simulink model "robio_auv5dof2017b"  (R2018b)
settings: Solver=VariableStepAuto  StartTime=0.0  StopTime=8.0  RelTol=0.05
settings Model: Creator=aditya-ubuntu  LastModifiedBy=aditya-ubuntu
settings SolverCC: MaxConsecutiveMinStep=10  MinimalZcImpactIntegration=on
settings DebuggingCC: ReadBeforeWriteMsg=DisableAll  WriteAfterWriteMsg=DisableAll  WriteAfterReadMsg=DisableAll  MultiTaskDSMMsg=none  UnderSpecifiedDimensionMsg=error
settings ModelReferenceCC: UpdateModelReferenceTargets=IfOutOfDate
settings SFSimCC: SFSimEcho=off

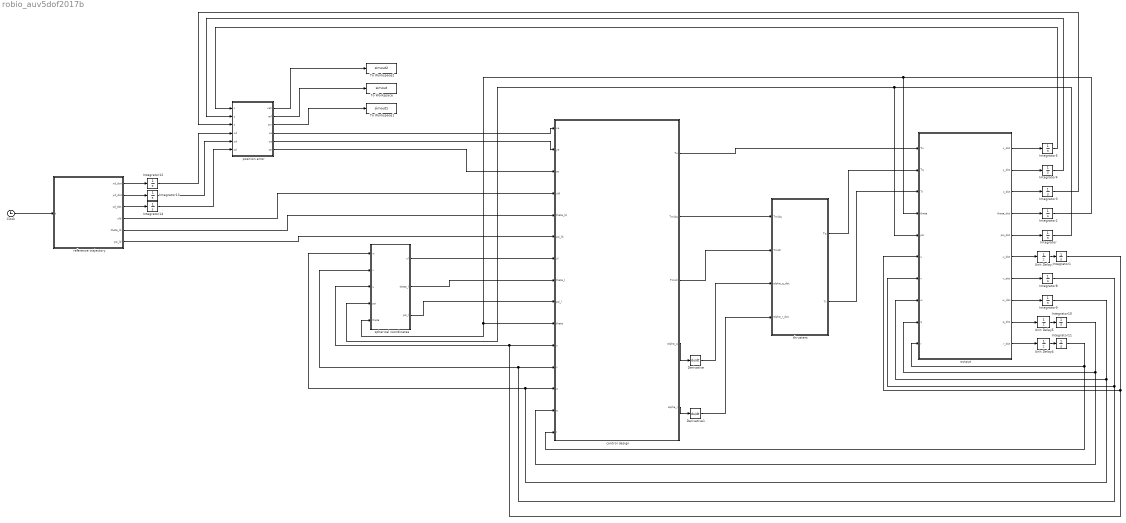
== system robio_auv5dof2017b ==
  Clock : Clock
      settings: Decimation=100
  Derivative : Derivative
  Derivative1 : Derivative
  Integrator{,2,4,8..9,12} (6 alike) : Integrator
  Integrator1 : Integrator  InitialCondition=0.3  AbsoluteTolerance=0.05
  Integrator10 : Integrator  InitialCondition=0.00001
  Integrator11 : Integrator  InitialCondition=0.0000001  AbsoluteTolerance=0.05
  Integrator13 : Integrator  InitialCondition=20
  Integrator14 : Integrator  InitialCondition=5
  Integrator3 : Integrator  InitialCondition=10
  Integrator5 : Integrator  InitialCondition=10
  To Workspace : ToWorkspace  VariableName=simout  SaveFormat=Timeseries  SampleTime=-1
  To Workspace1 : ToWorkspace  VariableName=simout1  SaveFormat=Timeseries  SampleTime=-1
  To Workspace2 : ToWorkspace  VariableName=simout2  SaveFormat=Timeseries  SampleTime=-1
  Unit Delay3 : UnitDelay  SampleTime=-1
  Unit Delay4 : UnitDelay  SampleTime=-1
  Unit Delay5 : UnitDelay  SampleTime=-1
  control design : MATLAB Function  TreatAsAtomicUnit=on
  output : MATLAB Function  TreatAsAtomicUnit=on
  position error : MATLAB Function  TreatAsAtomicUnit=on
  reference trajectory : MATLAB Function  TreatAsAtomicUnit=on
  spherical coordinates : MATLAB Function  TreatAsAtomicUnit=on
  thrusters : MATLAB Function  TreatAsAtomicUnit=on
  wires:
  output/1(x_dot) -> Integrator5/1
  output/2(y_dot) -> Integrator4/1
  output/3(z_dot) -> Integrator3/1
  output/4(theta_dot) -> Integrator2/1
  output/5(psi_dot) -> Integrator/1
  output/6(u_dot) -> Unit Delay3/1
  Integrator5/1 -> position error/1(x)
  Integrator4/1 -> position error/2(y)
  output/7(v_dot) -> Integrator8/1
  output/8(w_dot) -> Integrator9/1
  output/9(q_dot) -> Unit Delay5/1
  Integrator10/1 -> output/9(q), control design/14(q)
  Integrator9/1 -> output/8(w), spherical coordinates/1(w), control design/13(w)
  Integrator8/1 -> output/7(v), spherical coordinates/2(v), control design/12(v)
  Integrator1/1 -> output/6(u), spherical coordinates/3(u), control design/11(u)
  Integrator/1 -> output/5(psi), spherical coordinates/4(psi)
  Integrator2/1 -> output/4(theta), spherical coordinates/5(theta), control design/10(theta)
  Integrator11/1 -> control design/15(r), output/10(r)
  spherical coordinates/2(theta_l) -> control design/8(theta_l)
  spherical coordinates/3(psi_l) -> control design/9(psi_l)
  spherical coordinates/1(ul) -> control design/7(ul)
  reference trajectory/4(uld) -> control design/4(uld)
  Integrator3/1 -> position error/3(z)
  Unit Delay3/1 -> Integrator1/1
  Unit Delay4/1 -> Integrator11/1
  output/10(r_dot) -> Unit Delay4/1
  position error/6(ze) -> control design/3(ze)
  reference trajectory/1(xd_dot) -> Integrator12/1
  reference trajectory/2(yd_dot) -> Integrator13/1
  reference trajectory/3(zd_dot) -> Integrator14/1
  position error/5(ye) -> control design/2(ye)
  Integrator13/1 -> position error/5(yd)
  Integrator12/1 -> position error/4(xd)
  Integrator14/1 -> position error/6(zd)
  Unit Delay5/1 -> Integrator10/1
  position error/2(ref) -> To Workspace/1
  position error/3(err) -> To Workspace1/1
  position error/4(xe) -> control design/1(xe)
  position error/1(veh) -> To Workspace2/1
  reference trajectory/5(theta_ld) -> control design/5(theta_ld)
  reference trajectory/6(psi_ld) -> control design/6(psi_ld)
  Clock/1 -> reference trajectory/1(t)
  control design/2(Tmidq) -> thrusters/1(Tmidq)
  control design/3(Tmidr) -> thrusters/2(Tmidr)
  control design/4(alpha_q) -> Derivative/1
  control design/5(alpha_r) -> Derivative1/1
  thrusters/1(Tq) -> output/2(Tq)
  thrusters/2(Tr) -> output/3(Tr)
  Derivative/1 -> thrusters/3(alpha_q_dot)
  Derivative1/1 -> thrusters/4(alpha_r_dot)
  control design/1(Tu) -> output/1(Tu)

== matlab function robio_auv5dof2017b/thrusters ==
  data: Tq output; Tr output; Tmidq input; Tmidr input; alpha_q_dot input; alpha_r_dot input
function [Tq, Tr] = fcn(Tmidq, Tmidr, alpha_q_dot, alpha_r_dot)

    m5 = 22.5;
    m6 = 15.0;
    
%     disp('Tmidq');
%     disp(Tmidq);
%     disp('Tmidr');
%     disp(Tmidr);
%     disp('alpha_q_dot');
%     disp(alpha_q_dot);
%     disp('alpha_r_dot');
%     disp(alpha_r_dot);
    
    Tq = m5*( Tmidq + alpha_q_dot);
    
    disp("Tq");
    disp(Tq);
    
    Tr = m6*( Tmidr + alpha_r_dot);
    
    disp("Tr");
    disp(Tr);
       
end

== matlab function robio_auv5dof2017b/control design ==
  data: Tu output; Tmidq output size=6; Tmidr output; xe input; ye input size=3; ze input; uld input; theta_ld input; psi_ld input; ul input; theta_l input; psi_l input; theta input; u input; v input; w input; q input; r input; alpha_q output; alpha_r output
function [Tu, Tmidq, Tmidr, alpha_q, alpha_r] = controlinputfn5dof(xe, ye, ze, uld, theta_ld, psi_ld, ul, theta_l, psi_l, theta, u, v, w, q, r)
    
    gamma_r = 1.2;
    gamma_q = 1.2;
    gamma_u = 1;
    gamma_psi = 0.6;
    gamma_theta = 0.6;
    gamma_re = 1.2;
    
    k_psi = 0.5;
    k_theta = 0.5;
    k_u = 12;
    k_r = 0.9;
    k_q = 0.9;
    c_theta = 0.5;
    c_u = 12;
    
    m = [ 25.0 17.5 30.0 1.0 22.5 15.0 ];
    onebym = [1/25.0 1/17.5 1/30.0 1.0 1/22.5 1/15.0];
    row_g_invtri_Gml = 5.0;
    
    fu = (m(2)*v*r*onebym(1)) - (m(3)*w*q*onebym(1));    
    fv = (-(m(1)*u*r*onebym(2)));    
    fw = (m(1)*u*q*onebym(3));    
    fq = ((m(3)-m(1))*u*w*onebym(5)) - ((row_g_invtri_Gml)*onebym(5)*sin(theta));    
    fr = (m(1)-m(2))*u*v*onebym(6);
    
    disp('xe');
    disp(xe);
    disp('ye');
    disp(ye);
    disp('ze');
    disp(ze);
    
    re = sqrt(xe^2 + ye^2 + ze^2);
    
    disp('re');
    disp(re);
    xe_dot = uld*cos(theta_ld)*cos(psi_ld) - ul*cos(theta_l)*cos(psi_l);
    ye_dot = uld*cos(theta_ld)*sin(psi_ld) - ul*cos(theta_l)*sin(psi_l);
    ze_dot = -uld*sin(theta_ld) + ul*sin(theta_l);
    
    disp('xe_dot');
    disp(xe_dot);
    disp('ye_dot');
    disp(xe_dot);
    disp('ze_dot');
    disp(xe_dot);

    theta_a = atan2(w,sqrt(u^2 + v^2));
    theta_b = atan2( ze, sqrt(xe^2 + ye^2) );
    theta_le = theta_b - theta_l;
   
    psi_a = atan2(v,u);
    psi_b = atan2(ye,xe);
    psi_le = psi_b - psi_l;
    
    epower = e^(-c_theta*re);
    
    angle_in = (theta_ld - theta_b)*epower;
    
    uld_m = uld + c_u*re*cos(angle_in);
        
    theta_ld_m = theta_b + angle_in;
    
    re_dot = uld*{ cos(theta_ld)*cos(theta_b) + sin(theta_ld)*sin(theta_b)} - ul*{ cos(theta_l)*cos(theta_b)*cos(psi_le) + sin(theta_l)*sin(theta_b) };
    
    theta_b_dot = ((xe^2 + ye^2)*ze_dot - ze*(xe*xe_dot + ye*ye_dot)) / (re*re*sqrt(xe^2+ye^2));
    
    uld_m_dot = c_u*re_dot*cos(angle_in) - {c_u*re*epower*(theta_b*c_theta*re*re_dot - theta_b_dot)*sin(angle_in)};
    
    theta_ld_m_dot = theta_b_dot*(1 - epower) - c_theta*re*angle_in;
    
    ule = uld_m - ul;
    
    psi_b_dot = ( xe*ye_dot - ye*xe_dot ) / ( xe^2 + ye^2 );
    
    % duc*T is ignored
    Tu = m(1)*sec(theta_a)*sec(psi_a)*{ gamma_u^(-1)*{ k_u*ule + re*cos(theta_ld_m - theta_b)} +  uld_m_dot - fv*cos(theta_a)*sin(psi_a) - fw*sin(theta_a) };
    disp("Tu");
    disp(Tu);
    
    theta_leby2 = theta_le/2;
    theta_leby2_inv = 2/theta_le;
    theta_frac = (theta_ld_m + theta_l)/2;
    
    % dqc*T is ignored
    alpha_q_part1 = gamma_theta^(-1)*{ k_theta*theta_le - gamma_re^(-1)*re*ul*sin(theta_frac - theta_b)*sin(theta_leby2)*(theta_leby2_inv) };       
    alpha_q_part2 = theta_ld_m_dot + ( fw*(u^2 + v^2) - w*u*(fu + m(1)*Tu) + v*fv )/( ul*sqrt(u^2 + v^2) );    
    alpha_q = alpha_q_part1 + alpha_q_part2;
    disp('alpha_q');
    disp(alpha_q);
    eq = alpha_q - q;
    
    % drc*T is ignored
    alpha_r = cos(theta)*{ gamma_psi^(-1)*k_psi*psi_le + psi_b_dot - ( (u*fu - v(fu + m(1)*Tu))/ (u^2+v^2) ) };
    disp('alpha_r');
    disp(alpha_r);
    er = alpha_r - r;
    
   
    Tmidq = gamma_q^(-1)*(k_q*eq - gamma_theta*theta_le) - fq;
    disp("Tq");
    disp(Tq);
        
    Tmidr = gamma_r^(-1)*(k_r*er - gamma_psi*psi_le*sec(theta)) - fr;
    disp("Tr");
    disp(Tr);    

    
end

== matlab function robio_auv5dof2017b/output ==
  settings: updateMethod=DISCRETE
  data: x_dot output; y_dot output; z_dot output; theta_dot output; psi_dot output; u_dot output; v_dot output; w_dot output; q_dot output; r_dot output; Tu input; Tq input; Tr input; theta input; psi input; u input; v input; w input; q input; r input
function [ x_dot, y_dot, z_dot, theta_dot, psi_dot, u_dot, v_dot, w_dot, q_dot, r_dot] = outputfn5dof(Tu, Tq, Tr, theta, psi, u, v, w, q, r)
    

    m = [ 25.0 17.5 30.0 1.0 22.5 15.0 ];

    onebym = [1/25.0 1/17.5 1/30.0 1.0 1/22.5 1/15.0];
    
    du = 0; %0.6848;  (1-2rand)
    dv = 0; %0.2054; % 0.3(1-2rand)
    dw = 0; %0.2054; % 0.3(1-2rand)
    dq = 0; %0.1370; % 0.2(1-2rand)
    dr = 0; %0.1370; % 0.2(1-2rand)
    
    row_g_invtri_Gml = 5.0;
   
    fu = (m(2)*v*r*onebym(1)) - (m(3)*w*q*onebym(1));
    
    fv = (-(m(1)*u*r*onebym(2)));
    
    fw = (m(1)*u*q*onebym(3));
    
    fq = ((m(3)-m(1))*u*w*onebym(5)) - ((row_g_invtri_Gml)*onebym(5)*sin(theta));
    
    fr = (m(1)-m(2))*u*v*onebym(6);
    
    x_dot = u*cos(theta)*cos(psi) - v*sin(psi) + w*sin(theta)*cos(psi);
    
    y_dot = u*cos(theta)*sin(psi) + v*cos(psi) + w*sin(theta)*sin(psi);
    
    z_dot = -u*sin(theta) + w*cos(theta);
    
    theta_dot = q;
    
    psi_dot = r*sec(theta);
    
    u_dot = fu - onebym(1)*Tu - du*u*onebym(1);
    
    v_dot = fv - dv*onebym(2)*v;
    
    w_dot = fw - dw*onebym(3)*w;
    
    q_dot = fq + onebym(5)*Tq - dq*onebym(5)*q;
    
    r_dot = fr + onebym(6)*Tr - dr*onebym(6)*r; 
    
end

== matlab function robio_auv5dof2017b/reference trajectory ==
  data: xd_dot output; yd_dot output; zd_dot output; uld output; theta_ld output; psi_ld output; t input
function [xd_dot,yd_dot,zd_dot,uld,theta_ld,psi_ld] = fcn(t)
    
    uld = 1.5;
    psi_ld = 0;
    
    if( t<= 90)        
        theta_ld = 0;
        
    else
        theta_ld = -10;
    end
    
    xd_dot = uld*cos(theta_ld)*cos(psi_ld);
    
    yd_dot = uld*cos(theta_ld)*sin(psi_ld);
    
    zd_dot = -uld*sin(theta_ld);

end

== matlab function robio_auv5dof2017b/spherical coordinates ==
  data: w input; v input; u input; psi input; theta input; ul output; theta_l output; psi_l output
 function [ul, theta_l, psi_l] = sphericalfcn(w,v,u,psi,theta)
    
    ul = sqrt(u^2 + v^2 + w^2);
      
    %% CHECK
    

    theta_l = theta - atan2(w,sqrt(u^2 + v^2));
    
    psi_l = psi + atan2(y,u); 

    %%DISPLAY
    disp('u');
    disp(u);
    
    disp('v');
    disp(v);
    
    disp('w');
    disp(w);
    
    disp('ul');
    disp(ul);
    disp('theta_l');
    disp(theta_l);
    disp('psi_l');
    disp(psi_l);
end

== matlab function robio_auv5dof2017b/position error ==
  data: x input; y input; z input; veh output; ref output; err output; xe output; ye output; ze output; xd input; yd input; zd input

function [veh,ref,err,xe,ye,ze] = fcn(x,y,z,xd,yd,zd)
    xe = xd - x;
    
    ye = yd - y;
    
    ze = zd - z;
    
    veh = [x,y,z]';
    
    ref = [xd,yd,zd]';
    
    err = [xe,ye,ze]';
end
